simulink model "satellite_sim"  (R2018b)
settings: Solver=ode45  StartTime=0.0  StopTime=300  RelTol=1e-3  EnableMultiTasking=on
InitFcn:
  | addpath ./..
  | satelliteParam
  | satelliteParamHW8
undefined symbols (not defined in the file or in its folder): P, satellite_animation, satellite_ctrl
settings Model: Creator=beard  LastModifiedBy=beard
settings DataIOCC: LimitDataPoints=on  SaveFormat=Array  SignalLoggingSaveFormat=ModelDataLogs
settings OptimizationCC: ExpressionDepthLimit=2147483647  InitFltsAndDblsToZero=on  LifeSpan=inf
settings DebuggingCC: UnderspecifiedInitializationDetection=Classic  MergeDetectMultiDrivingBlocksExec=none  SolverPrmCheckMsg=warning  FcnCallInpInsideContextMsg=warning  StateNameClashWarn=warning  SFUnexpectedBacktrackingDiag=warning  SFNoUnconditionalDefaultTransitionDiag=warning  SFExecutionAtInitializationDiag=none
settings HardwareCC: ProdBitPerPointer=32  ProdBitPerSizeT=32  ProdBitPerPtrDiffT=32  ProdLargestAtomicFloat=None  ProdIntDivRoundTo=Undefined  ProdEndianess=Unspecified  ProdWordSize=32  ProdHWDeviceType=32-bit Generic
settings ModelReferenceCC: PropagateSignalLabelsOutOfModel=off
settings SFSimCC: SimUseLocalCustomCode=off
settings RTWCC: RTWUseLocalCustomCode=off
settings CodeAppCC: StateflowObjectComments=on
settings GRTTargetCC: TargetLangStandard=C89/C90 (ANSI)  GeneratePreprocessorConditionals=Disable all  CombineOutputUpdateFcns=off  GRTInterface=on
settings ConfigComp: CovMetricSettings=dw  CovHtmlReporting=on  CovSaveCumulativeToWorkspaceVar=on  CovSaveSingleToWorkspaceVar=on  CovExternalEMLEnable=off

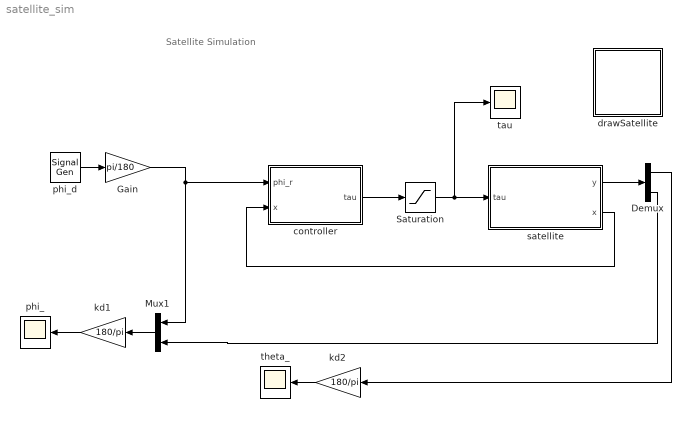
== system satellite_sim ==
  note: Satellite Simulation
  Demux : Demux  Outputs=2
  Gain : Gain  Gain=pi/180
  Mux1 : Mux  Inputs=2
  Saturation : Saturate  UpperLimit=P.taumax  LowerLimit=-P.taumax
  controller : Subsystem
  drawSatellite : Subsystem
      mask Display: image(imread('tv.jpg'))
  kd1 : Gain  Gain=180/pi
  kd2 : Gain  Gain=180/pi
  phi_ : Scope
  phi_d : SignalGenerator  WaveForm=square  Amplitude=15  Frequency=.015
  satellite : Subsystem
  tau : Scope
  theta_ : Scope
  wires:
  satellite/1(y) -> Demux/1
  phi_d/1 -> Gain/1
  Saturation/1 -> satellite/1(tau), tau/1
  Demux/1 -> kd2/1
  controller/1(tau) -> Saturation/1
  Mux1/1 -> kd1/1
  kd1/1 -> phi_/1
  Demux/2 -> Mux1/2
  Gain/1 -> Mux1/1, controller/1(phi_r)
  kd2/1 -> theta_/1
  satellite/2(x) -> controller/2(x)

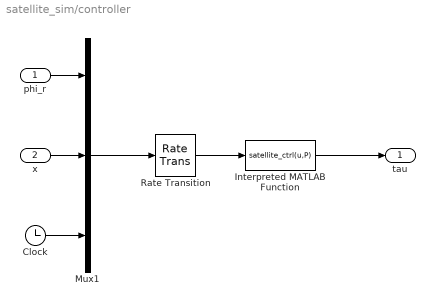
== system satellite_sim/controller ==
  phi_r : Inport
  x : Inport  Port=2
  Clock : Clock
  Interpreted MATLAB Function : MATLABFcn  MATLABFcn=satellite_ctrl(u,P)  OutputDimensions=1
  Mux1 : Mux  Inputs=3
  Rate Transition : RateTransition  OutPortSampleTime=P.Ts
  tau : Outport
  wires:
  Mux1/1 -> Rate Transition/1
  phi_r/1 -> Mux1/1
  Interpreted MATLAB Function/1 -> tau/1
  Clock/1 -> Mux1/3
  Rate Transition/1 -> Interpreted MATLAB Function/1
  x/1 -> Mux1/2

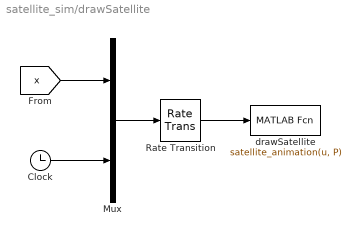
== system satellite_sim/drawSatellite ==
  Clock : Clock
  Mux : Mux  Inputs=2
  Rate Transition : RateTransition  OutPortSampleTime=P.t_plot
  drawSatellite : MATLABFcn  MATLABFcn=satellite_animation(u, P)  OutputDimensions=0
  wires:
  Rate Transition/1 -> drawSatellite/1
  Clock/1 -> Mux/2
  [x] -> Mux/1
  Mux/1 -> Rate Transition/1

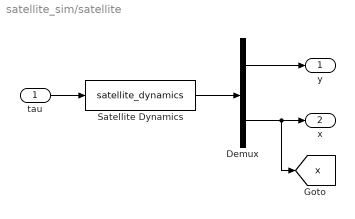
== system satellite_sim/satellite ==
  tau : Inport
  Demux : Demux  Outputs=[2;4]
  Satellite Dynamics : S-Function  FunctionName=satellite_dynamics  Parameters=P  SFunctionDeploymentMode=off  EnableBusSupport=off
  y : Outport
  x : Outport  Port=2
  tag scope: x=global
  wires:
  tau/1 -> Satellite Dynamics/1
  Satellite Dynamics/1 -> Demux/1
  Demux/1 -> y/1
  Demux/2 -> [x], x/1
